simulink model "ControllerSIRDQ"  (R2022b)
settings: Solver=ode14x  StartTime=t0  StopTime=t1  FixedStep=dt  RelTol=1e-6  AbsTol=1e-9
values from neighbouring files (symbols this model uses):
  beta1 = 1/3    (= 0.333333333333)    [MainCEoptCase4_FOPID.m]    (also in MainCEoptCase4_PID.m; MainGAoptCase4_FOPID.m; MainGAoptCase4_PID.m)
  gamma1 = 0.1    [MainCEoptCase4_FOPID.m]    (also in MainCEoptCase4_PID.m; MainGAoptCase4_FOPID.m; MainGAoptCase4_PID.m)
  gamma2 = 0.01    [MainCEoptCase4_FOPID.m]    (also in MainCEoptCase4_PID.m; MainGAoptCase4_FOPID.m; MainGAoptCase4_PID.m)
  Kd = x(3)    [MainCEoptCase4_FOPID.m]    (also in MainCEoptCase4_PID.m; MainGAoptCase4_FOPID.m; MainGAoptCase4_PID.m)
  Ki = x(2)    [MainCEoptCase4_FOPID.m]    (also in MainCEoptCase4_PID.m; MainGAoptCase4_FOPID.m; MainGAoptCase4_PID.m)
  Kp = x(1)    [MainCEoptCase4_FOPID.m]    (also in MainCEoptCase4_PID.m; MainGAoptCase4_FOPID.m; MainGAoptCase4_PID.m)
  N = 1000000    [MainCEoptCase4_FOPID.m]    (also in MainCEoptCase4_PID.m; MainGAoptCase4_FOPID.m; MainGAoptCase4_PID.m)
  tfinal = 60    [MainCEoptCase4_FOPID.m]    (also in MainCEoptCase4_PID.m; MainGAoptCase4_FOPID.m; MainGAoptCase4_PID.m)
  theta = 1/30    (= 0.0333333333333)    [MainCEoptCase4_FOPID.m]    (also in MainCEoptCase4_PID.m; MainGAoptCase4_FOPID.m; MainGAoptCase4_PID.m)
  tspan = t0:dt:t1    [MainCEoptCase4_FOPID.m]    (also in MainCEoptCase4_PID.m; MainGAoptCase4_FOPID.m; MainGAoptCase4_PID.m)
  tzero = 30    [MainCEoptCase4_FOPID.m]    (also in MainCEoptCase4_PID.m; MainGAoptCase4_FOPID.m; MainGAoptCase4_PID.m)
libraries: fod x2
settings Model: Creator=julio  LastModifiedBy=Ana Cláudia Rubim
settings SolverCC: AutoScaleAbsTol=off  AlgebraicLoopSolver=TrustRegion
settings DataIOCC: ReturnWorkspaceOutputs=off
settings OptimizationCC: LifeSpan=inf
settings DebuggingCC: UnconnectedInputMsg=warning  UnconnectedOutputMsg=warning  UnconnectedLineMsg=warning  SFUnexpectedBacktrackingDiag=warning  SFNoUnconditionalDefaultTransitionDiag=warning  SFMachineParentedDataDiag=warning  ArithmeticOperatorsInVariantConditions=warning
settings ModelReferenceCC: EnableRefExpFcnMdlSchedulingChecks=on
settings SFSimCC: SimUseLocalCustomCode=off  CustomCodeUndefinedFunction=UseInterfaceOnly
settings RTWCC: RTWUseLocalCustomCode=off
settings CodeAppCC: StateflowObjectComments=on
settings GRTTargetCC: TargetLangStandard=C89/C90 (ANSI)
settings ConfigComp: CovMetricSettings=dw  CovSaveCumulativeToWorkspaceVar=on  CovSaveSingleToWorkspaceVar=on  CovExternalEMLEnable=off

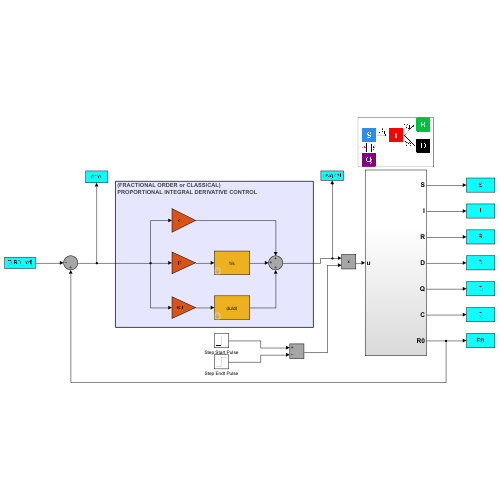
[thumbnail: Simulink's stored preview of the top-level diagram]
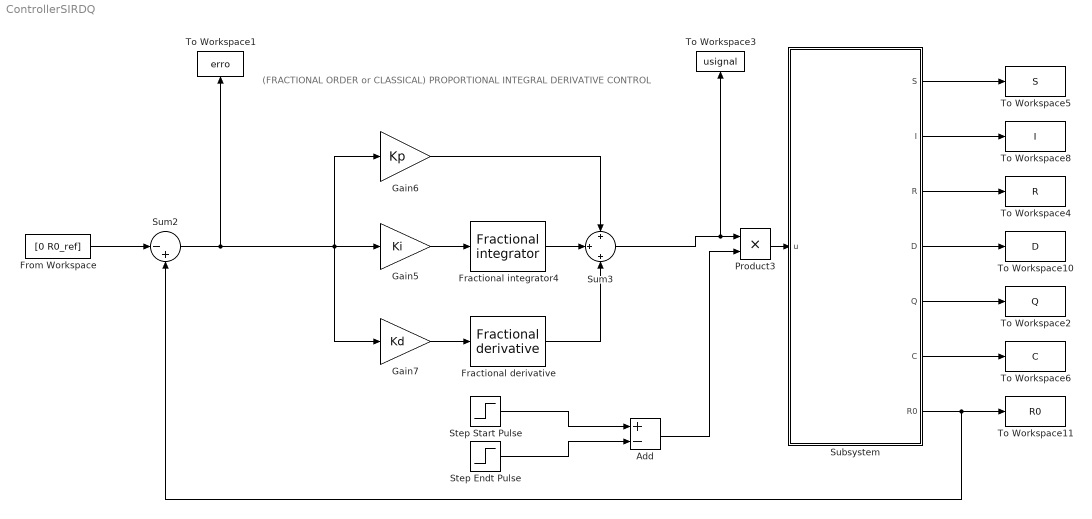
== system ControllerSIRDQ ==
  note: (FRACTIONAL ORDER or CLASSICAL)
      | PROPORTIONAL INTEGRAL DERIVATIVE CONTROL
  Add : Sum  Inputs=+-
  Fractional derivative : fod/Fractional derivative  gam=OrderD  ww=[0.001; 1000]  n=5  nFod=off
      settings: SourceProductName=FOMCON Toolbox
  Fractional integrator4 : fod/Fractional integrator  gam=OrderI  ww=[0.001; 1000]  n=5  nFod=off
      settings: SourceProductName=FOMCON Toolbox
  From Workspace : FromWorkspace  VariableName=[0 R0_ref]  OutDataTypeStr=double
  Gain5 : Gain  Gain=Ki
  Gain6 : Gain  Gain=Kp
  Gain7 : Gain  Gain=Kd
  Product3 : Product
  Step Endt Pulse : Step  Time=tspan(1,tfinal+1)  SampleTime=1
  Step Start Pulse : Step  Time=tspan(1,tzero+1)  SampleTime=1
  Subsystem : Subsystem
  Sum2 : Sum  Inputs=|-+
  Sum3 : Sum  Inputs=+|+|+
  To Workspace1 : ToWorkspace  VariableName=erro  SampleTime=-1
  To Workspace10 : ToWorkspace  VariableName=D  SampleTime=-1
  To Workspace11 : ToWorkspace  VariableName=R0  SampleTime=-1
  To Workspace2 : ToWorkspace  VariableName=Q  SampleTime=-1
  To Workspace3 : ToWorkspace  VariableName=usignal  SampleTime=-1
  To Workspace4 : ToWorkspace  VariableName=R  SampleTime=-1
  To Workspace5 : ToWorkspace  VariableName=S  SampleTime=-1
  To Workspace6 : ToWorkspace  VariableName=C  SampleTime=-1
  To Workspace8 : ToWorkspace  VariableName=I  SampleTime=-1
  wires:
  Subsystem/1(S) -> To Workspace5/1
  Subsystem/3(R) -> To Workspace4/1
  Subsystem/2(I) -> To Workspace8/1
  Subsystem/4(D) -> To Workspace10/1
  Subsystem/5(Q) -> To Workspace2/1
  From Workspace/1 -> Sum2/1
  Subsystem/6(C) -> To Workspace6/1
  Subsystem/7(R0) -> Sum2/2, To Workspace11/1
  Fractional derivative/1 -> Sum3/3
  Sum2/1 -> Gain7/1, Gain5/1, Gain6/1, To Workspace1/1
  Gain7/1 -> Fractional derivative/1
  Fractional integrator4/1 -> Sum3/2
  Gain5/1 -> Fractional integrator4/1
  Gain6/1 -> Sum3/1
  Sum3/1 -> Product3/1, To Workspace3/1
  Add/1 -> Product3/2
  Step Start Pulse/1 -> Add/1
  Step Endt Pulse/1 -> Add/2
  Product3/1 -> Subsystem/1(u)

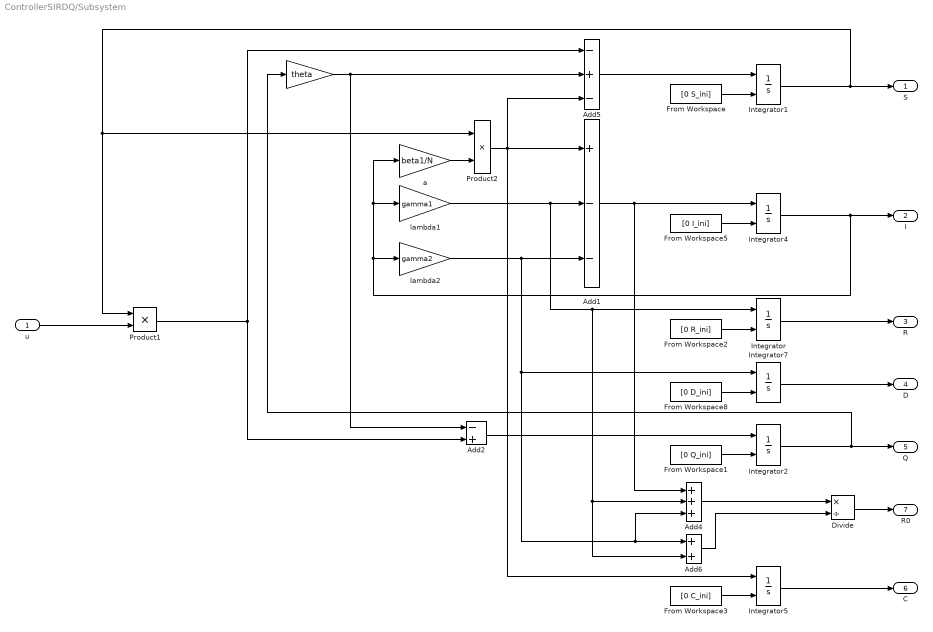
== system ControllerSIRDQ/Subsystem ==
  u : Inport
  "  " : Gain  Gain=theta
  Add1 : Sum  Inputs=+--
  Add2 : Sum  Inputs=-+
  Add4 : Sum  Inputs=+++
  Add5 : Sum  Inputs=-+-
  Add6 : Sum
  Divide : Product  Inputs=*/
  From Workspace : FromWorkspace  VariableName=[0 S_ini]  OutDataTypeStr=double
  From Workspace1 : FromWorkspace  VariableName=[0 Q_ini]
  From Workspace2 : FromWorkspace  VariableName=[0 R_ini]
  From Workspace3 : FromWorkspace  VariableName=[0 C_ini]
  From Workspace5 : FromWorkspace  VariableName=[0 I_ini]
  From Workspace8 : FromWorkspace  VariableName=[0 D_ini]
  Integrator{,2,4..5,7} (5 alike) : Integrator  InitialConditionSource=external
  Integrator1 : Integrator  InitialConditionSource=external  IgnoreLimit=on
  Product1 : Product
  Product2 : Product
  a : Gain  Gain=beta1/N
  lambda1 : Gain  Gain=gamma1
  lambda2 : Gain  Gain=gamma2
  S : Outport
  I : Outport  Port=2
  R : Outport  Port=3
  D : Outport  Port=4
  Q : Outport  Port=5
  C : Outport  Port=6
  R0 : Outport  Port=7
  wires:
  Integrator1/1 -> S/1, Product1/1, Product2/1
  From Workspace/1 -> Integrator1/2
  Integrator4/1 -> I/1, lambda1/1, a/1, lambda2/1
  From Workspace5/1 -> Integrator4/2
  Integrator/1 -> R/1
  From Workspace2/1 -> Integrator/2
  lambda1/1 -> Add6/2, Add4/2, Integrator/1, Add1/2
  From Workspace8/1 -> Integrator7/2
  lambda2/1 -> Add1/3, Add6/1, Add4/3, Integrator7/1
  Integrator7/1 -> D/1
  u/1 -> Product1/2
  a/1 -> Product2/2
  Add5/1 -> Integrator1/1
  "  "/1 -> Add2/1, Add5/2
  Product1/1 -> Add2/2, Add5/1
  From Workspace1/1 -> Integrator2/2
  Add2/1 -> Integrator2/1
  Integrator2/1 -> "  "/1, Q/1
  Product2/1 -> Add1/1, Integrator5/1, Add5/3
  Integrator5/1 -> C/1
  From Workspace3/1 -> Integrator5/2
  Add1/1 -> Integrator4/1, Add4/1
  Add4/1 -> Divide/1
  Add6/1 -> Divide/2
  Divide/1 -> R0/1
